simulink model "Modèle_système_pneumatique"  (R2023b)
settings: Solver=VariableStepAuto  StartTime=0.0  StopTime=10.0  RelTol=1e-3  AbsTol=1e-3
PreLoadFcn:
  | delta_p = 0.6; % MPa
  | p_init = 0.101325; % MPa
  | T_init = 293.15; % K
  | T_atm = 293.15; % K
  | 
  | A_valve_max = 4e-6; % m^2
  | A_valve_min = 1e-10; % m^2
  | 
  | A_pipe = 5e-6; % m^2
  | L_pipe = 1; % m
  | 
  | A_piston = 0.002; % m^2
  | L_piston = 0.2; % m
libraries: fl_lib x55, nesl_utility x7, simulink x1
(part 2 of 2)

== system Modèle_système_pneumatique/Atm ==
  Temperature Source : fl_lib/Thermal/Thermal Sources/Temperature Source  temperature=T_atm K
  T : PMIOPort  Side=Right
  connections:
  Temperature Source/LConn1 -- T/RConn1

== system Modèle_système_pneumatique/Atm1 ==
  Temperature Source : fl_lib/Thermal/Thermal Sources/Temperature Source  temperature=T_atm K
  T : PMIOPort  Side=Right
  connections:
  Temperature Source/LConn1 -- T/RConn1

== system Modèle_système_pneumatique/Atm2 ==
  Temperature Source : fl_lib/Thermal/Thermal Sources/Temperature Source  temperature=T_atm K
  T : PMIOPort  Side=Right
  connections:
  Temperature Source/LConn1 -- T/RConn1

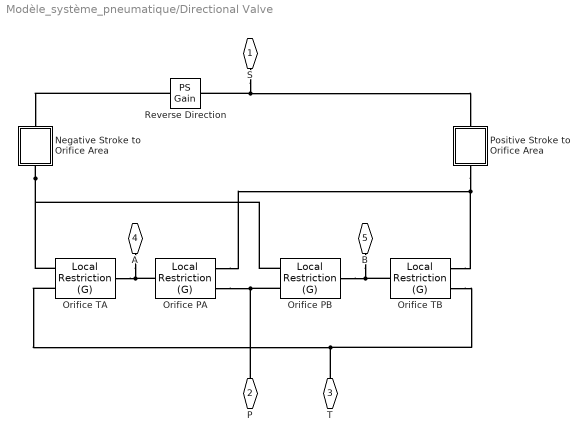
== system Modèle_système_pneumatique/Directional Valve ==
  Negative Stroke to Orifice Area : Subsystem
  Orifice PA : fl_lib/Gas/Elements/Local Restriction (G)  restriction_type=foundation.enum.restriction_type.variable  restriction_area=1e-3 m^2  min_area=A_leakage m^2  max_area=A_max m^2  area=A_port m^2  Cd=Cd  B_lam=0.999
      settings: InternalSimscapePortConfiguration="{\"Bottom\":[],\"Left\":[{\"id\":\"A\",\"label\":\"A\",\"type\":\"foundation.gas.gas\"},{\"id\":\"area_in\",\"label\":\"AR\",\"type\":\"input\"}],\"Right\":[{\"id\":\"B\",\"label\":\"B\",\"type\":\"foundation.gas.gas\"}],\"Top\":[]}"
  Orifice PB : fl_lib/Gas/Elements/Local Restriction (G)  restriction_type=foundation.enum.restriction_type.variable  restriction_area=1e-3 m^2  min_area=A_leakage m^2  max_area=A_max m^2  area=A_port m^2  Cd=Cd  B_lam=0.999
      settings: InternalSimscapePortConfiguration="{\"Bottom\":[],\"Left\":[{\"id\":\"A\",\"label\":\"A\",\"type\":\"foundation.gas.gas\"},{\"id\":\"area_in\",\"label\":\"AR\",\"type\":\"input\"}],\"Right\":[{\"id\":\"B\",\"label\":\"B\",\"type\":\"foundation.gas.gas\"}],\"Top\":[]}"
  Orifice TA : fl_lib/Gas/Elements/Local Restriction (G)  restriction_type=foundation.enum.restriction_type.variable  restriction_area=1e-3 m^2  min_area=A_leakage m^2  max_area=A_max m^2  area=A_port m^2  Cd=Cd  B_lam=0.999
      settings: InternalSimscapePortConfiguration="{\"Bottom\":[],\"Left\":[{\"id\":\"A\",\"label\":\"A\",\"type\":\"foundation.gas.gas\"},{\"id\":\"area_in\",\"label\":\"AR\",\"type\":\"input\"}],\"Right\":[{\"id\":\"B\",\"label\":\"B\",\"type\":\"foundation.gas.gas\"}],\"Top\":[]}"
  Orifice TB : fl_lib/Gas/Elements/Local Restriction (G)  restriction_type=foundation.enum.restriction_type.variable  restriction_area=1e-3 m^2  min_area=A_leakage m^2  max_area=A_max m^2  area=A_port m^2  Cd=Cd  B_lam=0.999
      settings: InternalSimscapePortConfiguration="{\"Bottom\":[],\"Left\":[{\"id\":\"A\",\"label\":\"A\",\"type\":\"foundation.gas.gas\"},{\"id\":\"area_in\",\"label\":\"AR\",\"type\":\"input\"}],\"Right\":[{\"id\":\"B\",\"label\":\"B\",\"type\":\"foundation.gas.gas\"}],\"Top\":[]}"
  Positive Stroke to Orifice Area : Subsystem
  Reverse Direction : fl_lib/Physical Signals/Functions/PS Gain  gain=-1
  S : PMIOPort  Side=Left
  P : PMIOPort  Port=2  Side=Left
  T : PMIOPort  Port=3  Side=Left
  A : PMIOPort  Port=4  Side=Right
  B : PMIOPort  Port=5  Side=Right
  connections:
  B/RConn1 -- Orifice TB/RConn1 -- Orifice PB/RConn1
  A/RConn1 -- Orifice PA/RConn1 -- Orifice TA/RConn1
  T/RConn1 -- Orifice TB/LConn1 -- Orifice TA/LConn1
  P/RConn1 -- Orifice PB/LConn1 -- Orifice PA/LConn1
  S/RConn1 -- Positive Stroke to Orifice Area/LConn1 -- Reverse Direction/LConn1
  Positive Stroke to Orifice Area/RConn1 -- Orifice TB/LConn2 -- Orifice PA/LConn2
  Negative Stroke to Orifice Area/RConn1 -- Orifice PB/LConn2 -- Orifice TA/LConn2
  Reverse Direction/RConn1 -- Negative Stroke to Orifice Area/LConn1

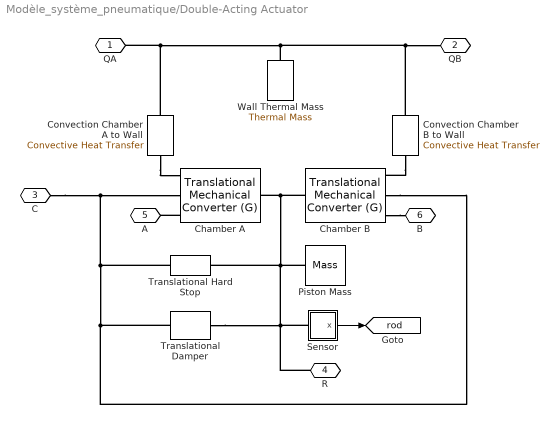
== system Modèle_système_pneumatique/Double-Acting Actuator ==
  Chamber A : fl_lib/Gas/Elements/Translational Mechanical Converter (G)  mech_orientation=simscape.enum.posneg.positive  displacement_spec=foundation.enum.DisplacementSpec.Calculate  length_init=x_init m  interface_area=A_piston m^2  dead_volume=0.1 * A_piston * x_max m^3  area_A=A_port m^2  environment_spec=foundation.enum.pressure_spec.atmospheric  environment_pressure=0.101325 MPa  p_I_specify=on  p_I_priority=High  p_I=p_init MPa  p_I_nominal_specify=off  p_I_nominal_unit=MPa  p_I_nominal_value=1  T_I_specify=on  T_I_priority=High  T_I=T_init K  T_I_nominal_specify=off  T_I_nominal_unit=K  T_I_nominal_value=1  rho_I_specify=off  rho_I_priority=None  rho_I=1.2 kg/m^3  rho_I_nominal_specify=off  rho_I_nominal_unit=kg/m^3  rho_I_nominal_value=1
      settings: InternalSimscapePortConfiguration="{\"Bottom\":[],\"Left\":[{\"id\":\"A\",\"label\":\"A\",\"type\":\"foundation.gas.gas\"},{\"id\":\"C\",\"label\":\"C\",\"type\":\"foundation.mechanical.translational.translational\"},{\"id\":\"H\",\"label\":\"H\",\"type\":\"foundation.thermal.thermal\"}],\"Right\":[{\"id\":\"R\",\"label\":\"R\",\"type\":\"foundation.mechanical.translational.translational\"}],\"Top\":[]}"
  Chamber B : fl_lib/Gas/Elements/Translational Mechanical Converter (G)  mech_orientation=simscape.enum.posneg.negative  displacement_spec=foundation.enum.DisplacementSpec.Calculate  length_init=- x_max + x_init m  interface_area=A_piston m^2  dead_volume=0.1 * A_piston * x_max m^3  area_A=A_port m^2  environment_spec=foundation.enum.pressure_spec.atmospheric  environment_pressure=0.101325 MPa  p_I_specify=on  p_I_priority=High  p_I=p_init MPa  p_I_nominal_specify=off  p_I_nominal_unit=MPa  p_I_nominal_value=1  T_I_specify=on  T_I_priority=High  T_I=T_init K  T_I_nominal_specify=off  T_I_nominal_unit=K  T_I_nominal_value=1  rho_I_specify=off  rho_I_priority=None  rho_I=1.2 kg/m^3  rho_I_nominal_specify=off  rho_I_nominal_unit=kg/m^3  rho_I_nominal_value=1
      settings: InternalSimscapePortConfiguration="{\"Bottom\":[],\"Left\":[{\"id\":\"A\",\"label\":\"A\",\"type\":\"foundation.gas.gas\"},{\"id\":\"C\",\"label\":\"C\",\"type\":\"foundation.mechanical.translational.translational\"},{\"id\":\"H\",\"label\":\"H\",\"type\":\"foundation.thermal.thermal\"}],\"Right\":[{\"id\":\"R\",\"label\":\"R\",\"type\":\"foundation.mechanical.translational.translational\"}],\"Top\":[]}"
  Convection Chamber A to Wall : fl_lib/Thermal/Thermal Elements/Convective Heat Transfer  thermal_type=foundation.enum.constant_variable.constant  area=2*A_piston + sqrt(pi*A_piston)*x_max m^2  heat_tr_coeff=heat_coeff W/(m^2 * K)  min_heat_tr_coeff=1e-3 W/(K*m^2)  T_specify=off  T_priority=None  T=0 K  T_nominal_specify=off  T_nominal_unit=K  T_nominal_value=1  Q_specify=off  Q_priority=None  Q=0 W  Q_nominal_specify=off  Q_nominal_unit=W  Q_nominal_value=1
  Convection Chamber B to Wall : fl_lib/Thermal/Thermal Elements/Convective Heat Transfer  thermal_type=foundation.enum.constant_variable.constant  area=2*A_piston + sqrt(pi*A_piston)*x_max m^2  heat_tr_coeff=heat_coeff W/(m^2 * K)  min_heat_tr_coeff=1e-3 W/(K*m^2)  T_specify=off  T_priority=None  T=0 K  T_nominal_specify=off  T_nominal_unit=K  T_nominal_value=1  Q_specify=off  Q_priority=None  Q=0 W  Q_nominal_specify=off  Q_nominal_unit=W  Q_nominal_value=1
  Piston Mass : fl_lib/Mechanical/Translational Elements/Mass  mass=M_piston kg  num_ports=foundation.enum.numPorts2.one  v_specify=off  v_priority=High  v=0 m/s  v_nominal_specify=off  v_nominal_unit=m/s  v_nominal_value=1  f_specify=off  f_priority=None  f=0 N  f_nominal_specify=off  f_nominal_unit=N  f_nominal_value=1
  Sensor : Subsystem
      mask Display: disp('S')
  Translational Damper : fl_lib/Mechanical/Translational Elements/Translational Damper  D=damp_mech N/(m/s)  v_specify=off  v_priority=None  v=0 m/s  v_nominal_specify=off  v_nominal_unit=m/s  v_nominal_value=1  f_specify=off  f_priority=None  f=0 N  f_nominal_specify=off  f_nominal_unit=N  f_nominal_value=1
  Translational Hard Stop : fl_lib/Mechanical/Translational Elements/Translational Hard Stop  upper_bnd=x_max m  lower_bnd=0 m  model=3  stiff_up=stiff_hard_stop N/m  stiff_low=stiff_hard_stop N/m  D_up=damp_hard_stop N/(m/s)  D_low=damp_hard_stop N/(m/s)  transition=0.1 mm  coeff_rest=0.7  v_tol=0.001 m/s  f_tol=0.001 N  v_specify=off  v_priority=None  v=0 m/s  v_nominal_specify=off  v_nominal_unit=m/s  v_nominal_value=1  f_specify=off  f_priority=None  f=0 N  f_nominal_specify=off  f_nominal_unit=N  f_nominal_value=1  x_specify=on  x_priority=High  x=x_init m  x_nominal_specify=off  x_nominal_unit=m  x_nominal_value=1  M_specify=off  M_priority=None  M=0
  Wall Thermal Mass : fl_lib/Thermal/Thermal Elements/Thermal Mass  mass_type=foundation.enum.constant_variable.constant  mass=M_actuator kg  sp_heat=cp J/kg/K  mass_min=1e-6 kg  num_ports=foundation.enum.numPorts2.one  m_specify=off  m_priority=High  m=1 kg  m_nominal_specify=off  m_nominal_unit=kg  m_nominal_value=1  T_specify=on  T_priority=High  T=T_init K  T_nominal_specify=off  T_nominal_unit=K  T_nominal_value=1  Q_specify=off  Q_priority=None  Q=0 W  Q_nominal_specify=off  Q_nominal_unit=W  Q_nominal_value=1
  QA : PMIOPort  Side=Left
  QB : PMIOPort  Port=2  Side=Right
  C : PMIOPort  Port=3  Side=Left
  R : PMIOPort  Port=4  Side=Right
  A : PMIOPort  Port=5  Side=Left
  B : PMIOPort  Port=6  Side=Right
  tag scope: rod=global
  wires:
  Sensor/1(x) -> [rod]
  connections:
  Chamber B/RConn1 -- R/RConn1 -- Sensor/LConn1 -- Translational Damper/LConn1 -- Piston Mass/LConn1 -- Translational Hard Stop/LConn1 -- Chamber A/RConn1
  Convection Chamber A to Wall/RConn1 -- QA/RConn1 -- Wall Thermal Mass/LConn1 -- Convection Chamber B to Wall/RConn1 -- QB/RConn1
  Translational Hard Stop/RConn1 -- Chamber B/LConn2 -- Translational Damper/RConn1 -- C/RConn1 -- Chamber A/LConn2
  Chamber A/LConn1 -- A/RConn1
  Chamber B/LConn1 -- B/RConn1
  Convection Chamber A to Wall/LConn1 -- Chamber A/LConn3
  Convection Chamber B to Wall/LConn1 -- Chamber B/LConn3

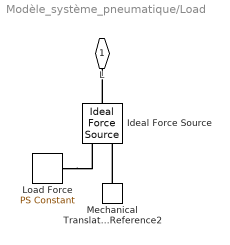
== system Modèle_système_pneumatique/Load ==
  Ideal Force Source : fl_lib/Mechanical/Mechanical Sources/Ideal Force Source
  Load Force : fl_lib/Physical Signals/Sources/PS Constant  constant=-500 N
  Mechanical Translational Reference2 : fl_lib/Mechanical/Translational Elements/Mechanical Translational Reference
  L : PMIOPort  Side=Right
  connections:
  Load Force/RConn1 -- Ideal Force Source/RConn1
  Mechanical Translational Reference2/LConn1 -- Ideal Force Source/RConn2
  Ideal Force Source/LConn1 -- L/RConn1

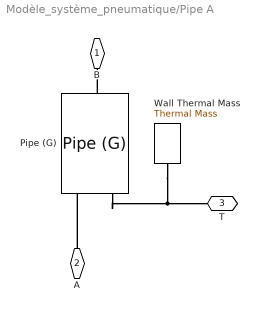
== system Modèle_système_pneumatique/Pipe A ==
  Pipe (G) : fl_lib/Gas/Elements/Pipe (G)  length=L_pipe m  area=A_pipe m^2  Dh=2*sqrt(A_pipe/pi) m  length_add=0.1 * L_pipe m  roughness=15e-6 m  Re_lam=2000  Re_tur=4000  shape_factor=64  Nu_lam=3.66  p_I_specify=on  p_I_priority=High  p_I=p_init MPa  p_I_nominal_specify=off  p_I_nominal_unit=MPa  p_I_nominal_value=1  T_I_specify=on  T_I_priority=High  T_I=T_init K  T_I_nominal_specify=off  T_I_nominal_unit=K  T_I_nominal_value=1  rho_I_specify=off  rho_I_priority=None  rho_I=1.2 kg/m^3  rho_I_nominal_specify=off  rho_I_nominal_unit=kg/m^3  rho_I_nominal_value=1
  Wall Thermal Mass : fl_lib/Thermal/Thermal Elements/Thermal Mass  mass_type=foundation.enum.constant_variable.constant  mass=rho_wall * A_pipe * L_pipe kg  sp_heat=cp_wall J/kg/K  mass_min=1e-6 kg  num_ports=foundation.enum.numPorts2.one  m_specify=off  m_priority=High  m=1 kg  m_nominal_specify=off  m_nominal_unit=kg  m_nominal_value=1  T_specify=on  T_priority=High  T=T_init K  T_nominal_specify=off  T_nominal_unit=K  T_nominal_value=1  Q_specify=off  Q_priority=None  Q=0 W  Q_nominal_specify=off  Q_nominal_unit=W  Q_nominal_value=1
  B : PMIOPort  Side=Right
  A : PMIOPort  Port=2  Side=Left
  T : PMIOPort  Port=3  Side=Left
  connections:
  Pipe (G)/RConn1 -- B/RConn1
  A/RConn1 -- Pipe (G)/LConn1
  Pipe (G)/LConn2 -- Wall Thermal Mass/LConn1 -- T/RConn1

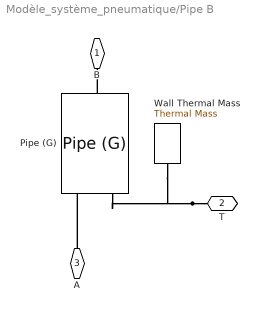
== system Modèle_système_pneumatique/Pipe B ==
  Pipe (G) : fl_lib/Gas/Elements/Pipe (G)  length=L_pipe m  area=A_pipe m^2  Dh=2*sqrt(A_pipe/pi) m  length_add=0.1 * L_pipe m  roughness=15e-6 m  Re_lam=2000  Re_tur=4000  shape_factor=64  Nu_lam=3.66  p_I_specify=on  p_I_priority=High  p_I=p_init MPa  p_I_nominal_specify=off  p_I_nominal_unit=MPa  p_I_nominal_value=1  T_I_specify=on  T_I_priority=High  T_I=T_init K  T_I_nominal_specify=off  T_I_nominal_unit=K  T_I_nominal_value=1  rho_I_specify=off  rho_I_priority=None  rho_I=1.2 kg/m^3  rho_I_nominal_specify=off  rho_I_nominal_unit=kg/m^3  rho_I_nominal_value=1
  Wall Thermal Mass : fl_lib/Thermal/Thermal Elements/Thermal Mass  mass_type=foundation.enum.constant_variable.constant  mass=rho_wall * A_pipe * L_pipe kg  sp_heat=cp_wall J/kg/K  mass_min=1e-6 kg  num_ports=foundation.enum.numPorts2.one  m_specify=off  m_priority=High  m=1 kg  m_nominal_specify=off  m_nominal_unit=kg  m_nominal_value=1  T_specify=on  T_priority=High  T=T_init K  T_nominal_specify=off  T_nominal_unit=K  T_nominal_value=1  Q_specify=off  Q_priority=None  Q=0 W  Q_nominal_specify=off  Q_nominal_unit=W  Q_nominal_value=1
  B : PMIOPort  Side=Right
  T : PMIOPort  Port=2  Side=Left
  A : PMIOPort  Port=3  Side=Left
  connections:
  T/RConn1 -- Wall Thermal Mass/LConn1 -- Pipe (G)/LConn2
  A/RConn1 -- Pipe (G)/LConn1
  Pipe (G)/RConn1 -- B/RConn1

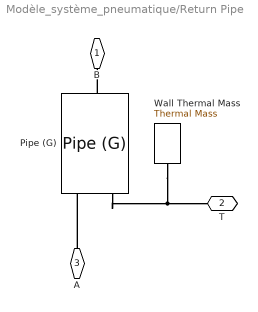
== system Modèle_système_pneumatique/Return Pipe ==
  Pipe (G) : fl_lib/Gas/Elements/Pipe (G)  length=L_pipe m  area=A_pipe m^2  Dh=2*sqrt(A_pipe/pi) m  length_add=0.1 * L_pipe m  roughness=15e-6 m  Re_lam=2000  Re_tur=4000  shape_factor=64  Nu_lam=3.66  p_I_specify=on  p_I_priority=High  p_I=p_init MPa  p_I_nominal_specify=off  p_I_nominal_unit=MPa  p_I_nominal_value=1  T_I_specify=on  T_I_priority=High  T_I=T_init K  T_I_nominal_specify=off  T_I_nominal_unit=K  T_I_nominal_value=1  rho_I_specify=off  rho_I_priority=None  rho_I=1.2 kg/m^3  rho_I_nominal_specify=off  rho_I_nominal_unit=kg/m^3  rho_I_nominal_value=1
  Wall Thermal Mass : fl_lib/Thermal/Thermal Elements/Thermal Mass  mass_type=foundation.enum.constant_variable.constant  mass=rho_wall * A_pipe * L_pipe kg  sp_heat=cp_wall J/kg/K  mass_min=1e-6 kg  num_ports=foundation.enum.numPorts2.one  m_specify=off  m_priority=High  m=1 kg  m_nominal_specify=off  m_nominal_unit=kg  m_nominal_value=1  T_specify=on  T_priority=High  T=T_init K  T_nominal_specify=off  T_nominal_unit=K  T_nominal_value=1  Q_specify=off  Q_priority=None  Q=0 W  Q_nominal_specify=off  Q_nominal_unit=W  Q_nominal_value=1
  B : PMIOPort  Side=Right
  T : PMIOPort  Port=2  Side=Left
  A : PMIOPort  Port=3  Side=Left
  connections:
  Pipe (G)/RConn1 -- B/RConn1
  A/RConn1 -- Pipe (G)/LConn1
  Pipe (G)/LConn2 -- Wall Thermal Mass/LConn1 -- T/RConn1

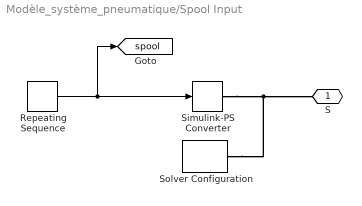
== system Modèle_système_pneumatique/Spool Input ==
  Repeating Sequence : simulink/Sources/Repeating Sequence  rep_seq_t=[0 1 1.2 3.8 4 6 6.2 8.8 9 10]  rep_seq_y=[0 0 5 5 0 0 -5 -5 0 0]
  Simulink-PS Converter : nesl_utility/Simulink-PS Converter  PhysicalDomain=network_engine_domain  SubClassName=ps_input  LeftPortType=input  RightPortType=output  PseudoPeriodic=off  Frequencies=[]  NoiseDistribution=none  NoiseParameters=[]  Unit=mm  AffineConversion=off  FilteringAndDerivatives=zero  SimscapeFilterOrder=1  InputFilterTimeConstant=0.001  UdotUserProvided=1
  Solver Configuration : nesl_utility/Solver Configuration  PhysicalDomain=network_engine_domain  SubClassName=solver  LeftPortType=input  RightPortType=generic  Tones=[]  Harmonics=[]  SimulateNoise=off  Profile=off  UseLocalSampling=off  EnableSwitchedLinearOptims=on  FrequencyDomain=off  UseCCode=off  RelTol=0.001  AbsTol=1e-06  MinStep=1e-09  ToWorkspace=off  RevertToSquareIcSolve=off  NumHomotopyIterations=100  PhasorMode=off  PhasorModeNumHarmonics=1  ConsistencySolver=NEWTON_XTOL_AFTER_FTOL  IndexReductionMethod=DerivativeReplacement  DoDC=off  ResidualTolerance=1e-9  ConsistencyTolSource=GLOBAL  ConsistencyAbsTol=0.001  ConsistencyRelTol=0.001  ConsistencyTolFactor=0.001  UseLocalSolver=off  LocalSolverChoice=NE_BACKWARD_EULER_ADVANCER  ResolveIndetEquations=on  FunctionEvalNumThread=1  LocalSolverSampleTime=0.001  DoFixedCost=off  MaxNonlinIter=3  MaxModeIter=2  ComputeImpulses=off  ImpulseIterations=2  LinearAlgebra=auto  LinearAlgebraNumThread=0  EquationFormulation=NE_TIME_EF  DelaysMemoryBudget=1024  AutomaticFiltering=on  FilteringTimeConstant=0.001  PartitionStorageMethod=AS_NEEDED  PartitionMemoryBudget=1024  PartitionMethod=FAST  MultibodyUseLocalSolver=off  MultibodyLocalSolverChoice=ODE1  MultibodyLocalSolverSampleTime=0.001
  S : PMIOPort  Side=Right
  tag scope: spool=global
  wires:
  Repeating Sequence/1 -> [spool], Simulink-PS Converter/1
  connections:
  Simulink-PS Converter/RConn1 -- S/RConn1 -- Solver Configuration/RConn1

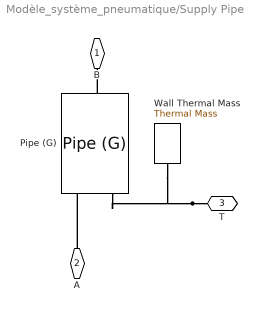
== system Modèle_système_pneumatique/Supply Pipe ==
  Pipe (G) : fl_lib/Gas/Elements/Pipe (G)  length=L_pipe m  area=A_pipe m^2  Dh=2*sqrt(A_pipe/pi) m  length_add=0.1 * L_pipe m  roughness=15e-6 m  Re_lam=2000  Re_tur=4000  shape_factor=64  Nu_lam=3.66  p_I_specify=on  p_I_priority=High  p_I=p_init MPa  p_I_nominal_specify=off  p_I_nominal_unit=MPa  p_I_nominal_value=1  T_I_specify=on  T_I_priority=High  T_I=T_init K  T_I_nominal_specify=off  T_I_nominal_unit=K  T_I_nominal_value=1  rho_I_specify=off  rho_I_priority=None  rho_I=1.2 kg/m^3  rho_I_nominal_specify=off  rho_I_nominal_unit=kg/m^3  rho_I_nominal_value=1
  Wall Thermal Mass : fl_lib/Thermal/Thermal Elements/Thermal Mass  mass_type=foundation.enum.constant_variable.constant  mass=rho_wall * A_pipe * L_pipe kg  sp_heat=cp_wall J/kg/K  mass_min=1e-6 kg  num_ports=foundation.enum.numPorts2.one  m_specify=off  m_priority=High  m=1 kg  m_nominal_specify=off  m_nominal_unit=kg  m_nominal_value=1  T_specify=on  T_priority=High  T=T_init K  T_nominal_specify=off  T_nominal_unit=K  T_nominal_value=1  Q_specify=off  Q_priority=None  Q=0 W  Q_nominal_specify=off  Q_nominal_unit=W  Q_nominal_value=1
  B : PMIOPort  Side=Right
  A : PMIOPort  Port=2  Side=Left
  T : PMIOPort  Port=3  Side=Left
  connections:
  T/RConn1 -- Wall Thermal Mass/LConn1 -- Pipe (G)/LConn2
  A/RConn1 -- Pipe (G)/LConn1
  Pipe (G)/RConn1 -- B/RConn1

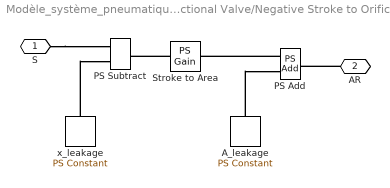
== system Modèle_système_pneumatique/Directional Valve/Negative Stroke to Orifice Area ==
  A_leakage : fl_lib/Physical Signals/Sources/PS Constant  constant=A_leakage m^2
  PS Add : fl_lib/Physical Signals/Functions/PS Add
  PS Subtract : fl_lib/Physical Signals/Functions/PS Subtract
  Stroke to Area : fl_lib/Physical Signals/Functions/PS Gain  gain=(A_max - A_leakage) / (x_max - x_leakage) m^2/m
  x_leakage : fl_lib/Physical Signals/Sources/PS Constant  constant=x_leakage m
  S : PMIOPort  Side=Left
  AR : PMIOPort  Port=2  Side=Right
  connections:
  S/RConn1 -- PS Subtract/LConn1
  PS Add/LConn1 -- Stroke to Area/RConn1
  Stroke to Area/LConn1 -- PS Subtract/RConn1
  A_leakage/RConn1 -- PS Add/LConn2
  x_leakage/RConn1 -- PS Subtract/LConn2
  AR/RConn1 -- PS Add/RConn1

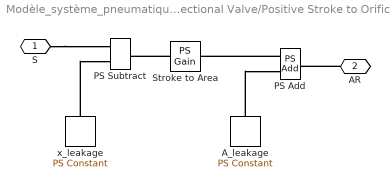
== system Modèle_système_pneumatique/Directional Valve/Positive Stroke to Orifice Area ==
  A_leakage : fl_lib/Physical Signals/Sources/PS Constant  constant=A_leakage m^2
  PS Add : fl_lib/Physical Signals/Functions/PS Add
  PS Subtract : fl_lib/Physical Signals/Functions/PS Subtract
  Stroke to Area : fl_lib/Physical Signals/Functions/PS Gain  gain=(A_max - A_leakage) / (x_max - x_leakage) m^2/m
  x_leakage : fl_lib/Physical Signals/Sources/PS Constant  constant=x_leakage m
  S : PMIOPort  Side=Left
  AR : PMIOPort  Port=2  Side=Right
  connections:
  AR/RConn1 -- PS Add/RConn1
  x_leakage/RConn1 -- PS Subtract/LConn2
  A_leakage/RConn1 -- PS Add/LConn2
  Stroke to Area/LConn1 -- PS Subtract/RConn1
  PS Add/LConn1 -- Stroke to Area/RConn1
  S/RConn1 -- PS Subtract/LConn1

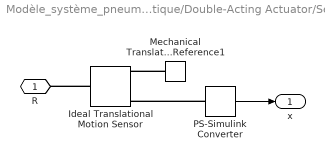
== system Modèle_système_pneumatique/Double-Acting Actuator/Sensor ==
  Ideal Translational Motion Sensor : fl_lib/Mechanical/Mechanical Sensors/Ideal Translational Motion Sensor  reference=foundation.enum.MeasurementReference.difference  acceleration_port=false  velocity_port=true  position_port=true  offset=0 m
  Mechanical Translational Reference1 : fl_lib/Mechanical/Translational Elements/Mechanical Translational Reference
  PS-Simulink Converter : nesl_utility/PS-Simulink Converter  PhysicalDomain=network_engine_domain  SubClassName=ps_output  LeftPortType=input  RightPortType=output  PseudoPeriodic=off  Frequencies=[]  VectorFormat=1-D array  Unit=m  AffineConversion=off
  R : PMIOPort  Side=Left
  x : Outport  VectorParamsAs1DForOutWhenUnconnected=off
  wires:
  PS-Simulink Converter/1 -> x/1
  connections:
  Mechanical Translational Reference1/LConn1 -- Ideal Translational Motion Sensor/RConn1
  Ideal Translational Motion Sensor/LConn1 -- R/RConn1
  PS-Simulink Converter/LConn1 -- Ideal Translational Motion Sensor/RConn3
